simulink model "SeparationForce_Drogue"  (R2024b)
settings: Solver=FixedStepAuto  StartTime=0.0  StopTime=10.0  FixedStep=0.001  RelTol=1e-3
values from neighbouring files (symbols this model uses):
  At_drogue = pi()*(d_reco_tube_inner_radius^2)    [separation.m]
  drogue_pressure = data{eventfilter("DROGUE"), "Air pressure"}    [SnatchForce.m]    (also in separation.m)
  gamma = 1.4    [separation.m]
  k_d = ea/Lh_drogue    (= 305.01246063)    [separation.m]
  Lh_drogue = Lh_drogue_e*0.3048    (= 15.24)    [separation.m]
  Vc_drogue = At_drogue*aft_length    [separation.m]
undefined symbols (not defined in the file or in its folder): mass
settings Model: Creator=Clare McMahon  LastModifiedBy=Clare McMahon

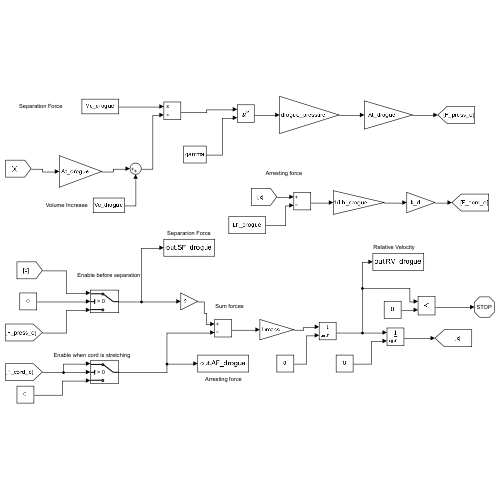
[thumbnail: Simulink's stored preview of the top-level diagram]
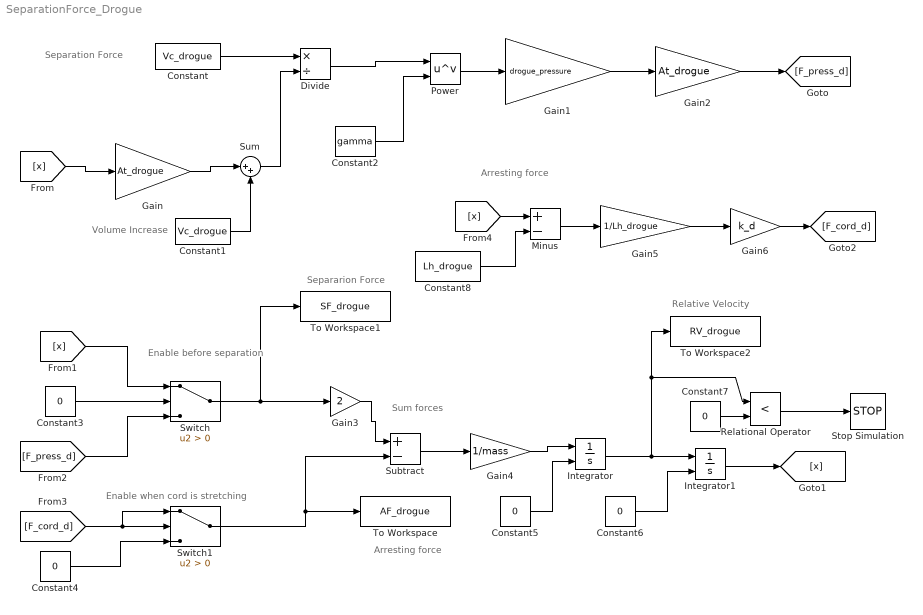
== system SeparationForce_Drogue ==
  note: Arresting force
  note: Relative Velocity
  note: Sum forces
  note: Arresting force
  note: Separarion Force
  note: Enable when cord is stretching
  note: Enable before separation
  note: Separation Force
  note: Volume Increase
  Constant : Constant  Value=Vc_drogue
  Constant1 : Constant  Value=Vc_drogue
  Constant2 : Constant  Value=gamma
  Constant{3..7} (5 alike) : Constant  Value=0
  Constant8 : Constant  Value=Lh_drogue
  Divide : Product  Inputs=*/
  Gain : Gain  Gain=At_drogue
  Gain1 : Gain  Gain=drogue_pressure
  Gain2 : Gain  Gain=At_drogue
  Gain3 : Gain  Gain=2
  Gain4 : Gain  Gain=1/mass
  Gain5 : Gain  Gain=1/Lh_drogue
  Gain6 : Gain  Gain=k_d
  Integrator : Integrator  InitialConditionSource=external
  Integrator1 : Integrator  InitialConditionSource=external
  Minus : Sum  Inputs=+-
  Power : Math  Operator=pow
  Relational Operator : RelationalOperator  Operator=<  OutDataTypeStr=boolean  RndMeth=Simplest  InputSameDT=off
  Stop Simulation : Stop
  Subtract : Sum  Inputs=+-
  Sum : Sum  Inputs=|++
  Switch : Switch  Criteria=u2 > Threshold  SaturateOnIntegerOverflow=off  InputSameDT=off
  Switch1 : Switch  Criteria=u2 > Threshold  SaturateOnIntegerOverflow=off  InputSameDT=off
  To Workspace : ToWorkspace  VariableName=AF_drogue  SaveFormat=Timeseries  SampleTime=-1
      settings: Save2DSignal=2-D array (concatenate along first dimension)
  To Workspace1 : ToWorkspace  VariableName=SF_drogue  SaveFormat=Timeseries  SampleTime=-1
      settings: Save2DSignal=2-D array (concatenate along first dimension)
  To Workspace2 : ToWorkspace  VariableName=RV_drogue  SaveFormat=Timeseries  SampleTime=-1
      settings: Save2DSignal=2-D array (concatenate along first dimension)
  wires:
  Constant/1 -> Divide/1
  Gain/1 -> Sum/1
  Constant1/1 -> Sum/2
  Sum/1 -> Divide/2
  Divide/1 -> Power/1
  Constant2/1 -> Power/2
  Power/1 -> Gain1/1
  Gain1/1 -> Gain2/1
  Gain2/1 -> [F_press_d]
  [x] -> Gain/1
  [x] -> Switch/1
  Constant3/1 -> Switch/2
  [F_press_d] -> Switch/3
  Switch/1 -> To Workspace1/1, Gain3/1
  [F_cord_d] -> Switch1/1, Switch1/2
  Constant4/1 -> Switch1/3
  Gain3/1 -> Subtract/1
  Switch1/1 -> To Workspace/1, Subtract/2
  Subtract/1 -> Gain4/1
  Gain4/1 -> Integrator/1
  Constant5/1 -> Integrator/2
  Constant6/1 -> Integrator1/2
  Integrator/1 -> To Workspace2/1, Relational Operator/1, Integrator1/1
  Constant7/1 -> Relational Operator/2
  Relational Operator/1 -> Stop Simulation/1
  Integrator1/1 -> [x]
  [x] -> Minus/1
  Constant8/1 -> Minus/2
  Minus/1 -> Gain5/1
  Gain5/1 -> Gain6/1
  Gain6/1 -> [F_cord_d]
